simulink model "Simulink_p_2"  (R2018b)
settings: Solver=VariableStepAuto  StartTime=0.0  StopTime=10.0  RelTol=1e-3
libraries: simulink_extras x1
settings Model: Creator=Alberto  LastModifiedBy=Alberto

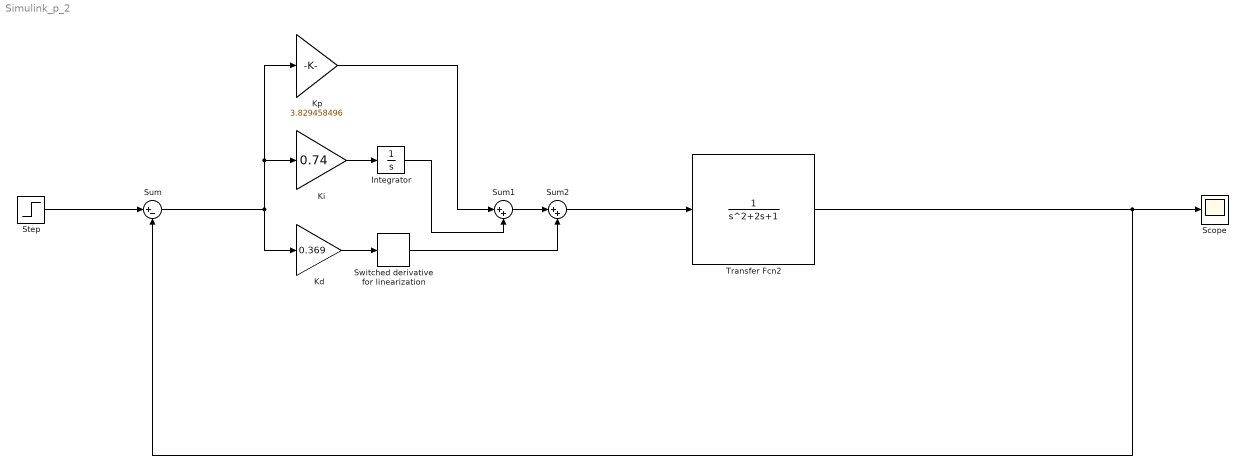
== system Simulink_p_2 ==
  Integrator : Integrator
  "Kd " : Gain  Gain=0.369
  "Ki " : Gain  Gain=0.74
  "Kp " : Gain  Gain=3.829458496
  Scope : Scope
  Step : Step  SampleTime=0
  Sum : Sum  Inputs=|+-
  Sum1 : Sum  Inputs=|++
  Sum2 : Sum  Inputs=|++
  Switched derivative for linearization : simulink_extras/Linearization/Switched derivative for linearization  switchVal=0  derivConst=100
      settings: SourceProductName=Simulink  SourceProductBaseCode=SL
  Transfer Fcn2 : TransferFcn
  wires:
  Step/1 -> Sum/1
  Sum/1 -> "Kd "/1, "Ki "/1, "Kp "/1
  "Ki "/1 -> Integrator/1
  "Kp "/1 -> Sum1/1
  Integrator/1 -> Sum1/2
  Switched derivative for linearization/1 -> Sum2/2
  Sum1/1 -> Sum2/1
  "Kd "/1 -> Switched derivative for linearization/1
  Transfer Fcn2/1 -> Sum/2, Scope/1
  Sum2/1 -> Transfer Fcn2/1
